simulink model "sampleModel2120"  (R2021a)
settings: Solver=VariableStepAuto  StartTime=0.0  StopTime=10.0  RelTol=1e-3
undefined symbols (not defined in the file or in its folder): DiscIntNeverNeededParam, magnitude, Newton, Raphson
libraries: simulink x67, pid_lib x12
(part 1 of 2)
settings Model: Creator=lenovo  LastModifiedBy=lenovo

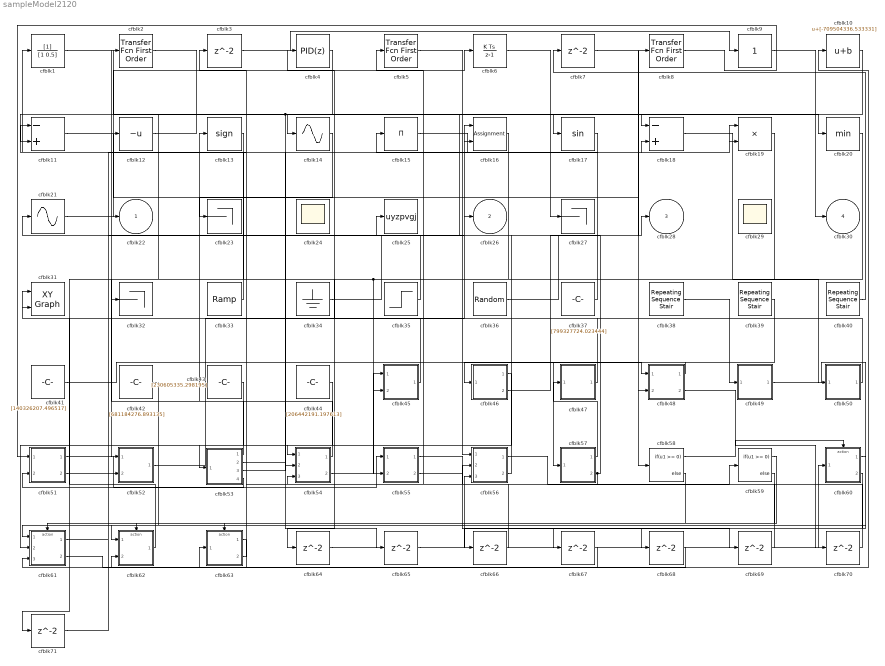
== system sampleModel2120 ==
  cfblk1 : DiscreteFilter  SampleTime=1
  cfblk10 : Bias  Bias=[-709504336.533331]
  cfblk11 : Sum  Inputs=-+
  cfblk12 : UnaryMinus
  cfblk13 : Signum
  cfblk14 : Sin  TimeSource=Use external signal  SampleTime=0
  cfblk15 : Product  Inputs=*
  cfblk16 : Assignment  DiagnosticForDimensions=Warning  IndexOptions=Index vector (dialog)  Indices=1  OutputSizes=1
  cfblk17 : Trigonometry
  cfblk18 : Sum  Inputs=-+
  cfblk19 : Product  Inputs=**
  cfblk2 : simulink/Discrete/Transfer Fcn First Order  PoleZ=0.95  ICPrevOutput=0.0  DoSatur=off
  cfblk20 : MinMax
  cfblk21 : Sin  TimeSource=Use external signal  SampleTime=0
  cfblk23 : Terminator
  cfblk24 : Scope
      settings: Floating=on
  cfblk25 : ToWorkspace  VariableName=uyzpvgj  SaveFormat=Timeseries  SampleTime=-1
  cfblk27 : Terminator
  cfblk29 : Scope
      settings: Floating=on
  cfblk{3,7,64..71} (10 alike) : Delay  SampleTime=1
  cfblk31 : simulink/Sinks/XY Graph  xmin=-1  xmax=1  ymin=-1  ymax=1  st=-1
  cfblk32 : Terminator
  cfblk33 : simulink/Sources/Ramp  slope=[-9170.423728]  start=[47.124759]  InitialOutput=[-914026.200250]
  cfblk34 : Ground
  cfblk35 : Step  Time=[9.000000]  Before=[-795213372.799819]  After=[478961987.281532]  SampleTime=0
  cfblk36 : RandomNumber  Mean=[10617.420643]  Variance=[21176.794349]  Seed=[230646429.000000]  SampleTime=0.1
  cfblk37 : Constant  Value=[799327724.023444]  SampleTime=1
  cfblk38 : simulink/Sources/Repeating Sequence Stair  OutValues=[-433408772.823916, -415254257.712957]  tsamp=-1  OutMin=[]  OutMax=[]  OutDataTypeStr=double  OutputDataTypeScalingMode=double  OutDataType=fixdt(0,8)  ConRadixGroup=Best Precision: Vector-wise  OutScaling=2^-12
  cfblk39 : simulink/Sources/Repeating Sequence Stair  OutValues=[-289850517.751217, -807875800.203243]  tsamp=-1  OutMin=[]  OutMax=[]  OutDataTypeStr=double  OutputDataTypeScalingMode=double  OutDataType=fixdt(0,8)  ConRadixGroup=Best Precision: Vector-wise  OutScaling=2^-12
  cfblk4 : pid_lib/PID Controller  Controller=PID  Form=Parallel  TimeDomain=Discrete-time  UseExternalTs=off  SampleTime=1  IntegratorMethod=Forward Euler  FilterMethod=Forward Euler  ControllerParametersSource=internal  P=1  I=1  D=0  UseFilter=on  N=100  TunerSelectOption=Transfer Function Based (PID Tuner App)  InitialConditionSource=internal  InitialConditionForIntegrator=0  InitialConditionForFilter=0  DifferentiatorICPrevScaledInput=0  ExternalReset=none  TrackingMode=off  Kt=1  LimitOutput=off  SatLimitsSource=internal  UpperSaturationLimit=inf  LowerSaturationLimit=-inf  LinearizeAsGain=off  AntiWindupMode=none  Kb=1  POutMin=[]  POutMax=[]  IOutMin=[]  IOutMax=[]  DOutMin=[]  DOutMax=[]  NOutMin=[]  NOutMax=[]  SumOutMin=[]  SumOutMax=[]  SaturationOutMin=[]  SaturationOutMax=[]  PParamMin=[]  PParamMax=[]  IParamMin=[]  IParamMax=[]  DParamMin=[]  DParamMax=[]  NParamMin=[]  NParamMax=[]  KbParamMin=[]  KbParamMax=[]  KtParamMin=[]  KtParamMax=[]  KbOutMin=[]  KbOutMax=[]  KtOutMin=[]  KtOutMax=[]  IntegratorOutMin=[]  IntegratorOutMax=[]  FilterOutMin=[]  FilterOutMax=[]  SumI1OutMin=[]  SumI1OutMax=[]  SumI2OutMin=[]  SumI2OutMax=[]  SumI3OutMin=[]  SumI3OutMax=[]  SumI4OutMin=[]  SumI4OutMax=[]  SumDOutMin=[]  SumDOutMax=[]  DifferentiatorOutMin=[]  DifferentiatorOutMax=[]  FilterDiffOutCoefMin=[]  FilterDiffOutCoefMax=[]  ReciprocalOutMin=[]  ReciprocalOutMax=[]  SumDenOutMin=[]  SumDenOutMax=[]  SumNumOutMin=[]  SumNumOutMax=[]  DivideOutMin=[]  DivideOutMax=[]  UdiffTsProdOutMin=[]  UdiffTsProdOutMax=[]  NTsProdOutMin=[]  NTsProdOutMax=[]  UintegralTsProdOutMin=[]  UintegralTsProdOutMax=[]  UngainTsProdOutMin=[]  UngainTsProdOutMax=[]  IntegratorContinuousStateAttributes=''  IntegratorStateMustResolveToSignalObject=off  IntegratorRTWStateStorageClass=Auto  FilterContinuousStateAttributes=''  FilterStateMustResolveToSignalObject=off  FilterRTWStateStorageClass=Auto  ParallelPVariant=InternalParameters  IdealPVariant=Disabled  IVariant=InternalParameters  DVariant=InternalParameters  IntegratorVariant=Discrete  SatVariant=Disabled  AWVariant=Passthrough  PCopyVariant=Disabled  TRVariant=Disabled  FdbkBlocksVariant=Forward  IdealPFdbkVariant=Disabled  SatFdbkVariant=Disabled  DerivativeFilterVariant=ForwardEulerFilter  NVariant=InternalParameters  NCopyVariant=Disabled  FilterICVariant=InternalICsFilter  IntegratorICVariant=InternalICs  ExternalResetVariant=Disabled  TRSumVariant=Passthrough  SumFdbkVariant=Disabled  SumVariant=Sum_PID  TsampFilterVariant=InternalTs  TsampNgainVariant=Passthrough  TsampIntegralVariant=Passthrough  ExternalSaturationOutDataTypeStr=Inherit: Same as second input
  cfblk40 : simulink/Sources/Repeating Sequence Stair  OutValues=[599228246.238422, -891664695.317547]  tsamp=-1  OutMin=[]  OutMax=[]  OutDataTypeStr=double  OutputDataTypeScalingMode=double  OutDataType=fixdt(0,8)  ConRadixGroup=Best Precision: Vector-wise  OutScaling=2^-12
  cfblk41 : Constant  Value=[140326207.496517]  SampleTime=1
  cfblk42 : Constant  Value=[681184276.893135]  SampleTime=1
  cfblk43 : Constant  Value=[230605335.298195]  SampleTime=1
  cfblk44 : Constant  Value=[206442191.197613]  SampleTime=1
  cfblk45 : Subsystem
  cfblk46 : Subsystem
  cfblk47 : Subsystem
  cfblk48 : Subsystem
  cfblk49 : Subsystem
  cfblk5 : simulink/Discrete/Transfer Fcn First Order  PoleZ=0.95  ICPrevOutput=0.0  DoSatur=off
  cfblk50 : Subsystem
  cfblk51 : Subsystem
  cfblk52 : Subsystem
  cfblk53 : Subsystem
  cfblk54 : Subsystem
  cfblk55 : Subsystem
  cfblk56 : Subsystem
  cfblk57 : Subsystem
  cfblk58 : If  IfExpression=u1 >= 0  SampleTime=1
  cfblk59 : If  IfExpression=u1 >= 0  SampleTime=1
  cfblk6 : DiscreteIntegrator  ICPrevOutput=DiscIntNeverNeededParam  ICPrevScaledInput=DiscIntNeverNeededParam
  cfblk60 : Subsystem  TreatAsAtomicUnit=on
  cfblk61 : Subsystem  TreatAsAtomicUnit=on
  cfblk62 : Subsystem  TreatAsAtomicUnit=on
  cfblk63 : Subsystem  TreatAsAtomicUnit=on
  cfblk8 : simulink/Discrete/Transfer Fcn First Order  PoleZ=0.95  ICPrevOutput=0.0  DoSatur=off
  cfblk9 : simulink/Math Operations/Slider Gain  gain=1  low=0  high=2
  cfblk22 : Outport
  cfblk26 : Outport  Port=2
  cfblk28 : Outport  Port=3
  cfblk30 : Outport  Port=4
  wires:
  cfblk1/1 -> cfblk14/1
  cfblk33/1 -> cfblk1/1
  cfblk52/1(cfblk2) -> cfblk16/1
  cfblk3/1 -> cfblk9/1
  cfblk49/1(cfblk2) -> cfblk61/1(cfblk1)
  cfblk44/1 -> cfblk54/1(cfblk1)
  cfblk21/1 -> cfblk6/1
  cfblk39/1 -> cfblk57/1(cfblk1)
  cfblk51/1(cfblk2) -> cfblk55/1(cfblk1)
  cfblk53/1(cfblk2) -> cfblk2/1
  cfblk45/1(cfblk2) -> cfblk31/1
  cfblk34/1 -> cfblk20/1
  cfblk8/1 -> cfblk51/1(cfblk1)
  cfblk54/1(cfblk2) -> cfblk13/1
  cfblk43/1 -> cfblk61/2(cfblk12)
  cfblk13/1 -> cfblk52/1(cfblk1)
  cfblk40/1 -> cfblk7/1
  cfblk18/1 -> cfblk50/1(cfblk1)
  cfblk12/1 -> cfblk17/1
  cfblk57/1(cfblk2) -> cfblk47/1(cfblk1)
  cfblk37/1 -> cfblk15/1
  cfblk9/1 -> cfblk30/1
  cfblk35/1 -> cfblk21/1
  cfblk14/1 -> cfblk23/1
  cfblk38/1 -> cfblk49/1(cfblk1)
  cfblk41/1 -> cfblk48/1(cfblk1)
  cfblk51/2(cfblk12) -> cfblk26/1
  cfblk57/2(cfblk17) -> cfblk22/1, cfblk54/3(cfblk11)
  cfblk46/1(cfblk2) -> cfblk53/1(cfblk1)
  cfblk7/1 -> cfblk58/1
  cfblk46/2(cfblk8) -> cfblk28/1
  cfblk42/1 -> cfblk62/1(cfblk1)
  cfblk61/1(cfblk2) -> cfblk19/1
  cfblk62/1(cfblk2) -> cfblk31/2
  cfblk16/1 -> cfblk45/2(cfblk15), cfblk71/1
  cfblk6/1 -> cfblk27/1
  cfblk50/1(cfblk2) -> cfblk3/1
  cfblk47/1(cfblk2) -> cfblk4/1
  cfblk36/1 -> cfblk8/1
  cfblk5/1 -> cfblk56/1(cfblk1)
  cfblk4/1 -> cfblk32/1
  cfblk15/1 -> cfblk19/2
  cfblk17/1 -> cfblk16/2
  cfblk61/2(cfblk14) -> cfblk10/1
  cfblk11/1 -> cfblk48/2(cfblk13)
  cfblk20/1 -> cfblk55/2(cfblk10)
  cfblk2/1 -> cfblk18/1
  cfblk53/3(cfblk6) -> cfblk18/2
  cfblk56/1(cfblk2) -> cfblk59/1
  cfblk10/1 -> cfblk11/2, cfblk54/2(cfblk10)
  cfblk63/1(cfblk2) -> cfblk61/3(cfblk13)
  cfblk56/2(cfblk12) -> cfblk25/1
  cfblk53/4(cfblk7) -> cfblk51/2(cfblk11)
  cfblk48/1(cfblk2) -> cfblk46/1(cfblk1)
  cfblk63/2(cfblk8) -> cfblk12/1
  cfblk54/2(cfblk12) -> cfblk45/1(cfblk1)
  cfblk58/1 -> cfblk60/Action
  cfblk58/2 -> cfblk61/Action
  cfblk59/1 -> cfblk62/Action
  cfblk59/2 -> cfblk63/Action
  cfblk19/1 -> cfblk64/1
  cfblk64/1 -> cfblk56/3(cfblk11)
  cfblk53/2(cfblk5) -> cfblk65/1
  cfblk65/1 -> cfblk60/1(cfblk1)
  cfblk60/1(cfblk2) -> cfblk66/1
  cfblk66/1 -> cfblk11/1
  cfblk60/2(cfblk14) -> cfblk67/1
  cfblk67/1 -> cfblk62/2(cfblk13)
  cfblk55/1(cfblk2) -> cfblk68/1
  cfblk68/1 -> cfblk63/1(cfblk1)
  cfblk55/2(cfblk11) -> cfblk69/1
  cfblk69/1 -> cfblk5/1
  cfblk48/2(cfblk14) -> cfblk70/1
  cfblk70/1 -> cfblk56/2(cfblk10)
  cfblk71/1 -> cfblk52/2(cfblk15)

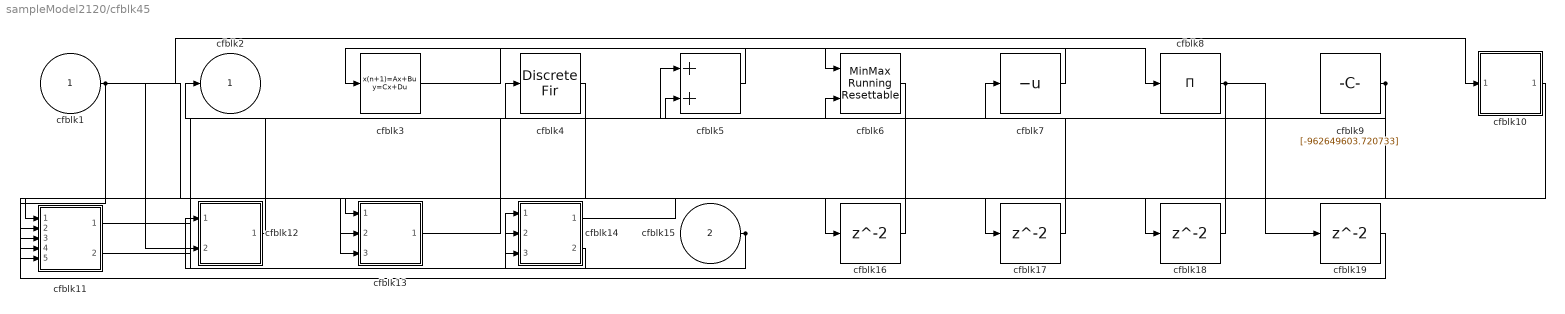
== system sampleModel2120/cfblk45 ==
  cfblk1 : Inport
  cfblk15 : Inport  Port=2
  cfblk10 : Subsystem
  cfblk11 : Subsystem
  cfblk12 : Subsystem
  cfblk13 : Subsystem
  cfblk14 : Subsystem
  cfblk{16..19} (4 alike) : Delay  SampleTime=1
  cfblk3 : DiscreteStateSpace
  cfblk4 : DiscreteFir  SampleTime=1
  cfblk5 : Sum
  cfblk6 : simulink/Math Operations/MinMax Running Resettable  Function=min  vinit=0.0
  cfblk7 : UnaryMinus
  cfblk8 : Product  Inputs=*
  cfblk9 : Constant  Value=[-962649603.720733]  SampleTime=1
  cfblk2 : Outport
  wires:
  cfblk5/1 -> cfblk3/1
  cfblk12/1(cfblk2) -> cfblk2/1
  cfblk7/1 -> cfblk6/1
  cfblk1/1 -> cfblk10/1(cfblk1), cfblk11/3(cfblk7), cfblk12/2(cfblk11), cfblk13/3(cfblk12)
  cfblk11/1(cfblk2) -> cfblk14/1(cfblk1)
  cfblk9/1 -> cfblk4/1, cfblk11/5(cfblk9)
  cfblk8/1 -> cfblk17/1, cfblk18/1, cfblk19/1
  cfblk3/1 -> cfblk8/1
  cfblk4/1 -> cfblk11/1(cfblk1)
  cfblk13/1(cfblk2) -> cfblk7/1
  cfblk6/1 -> cfblk11/2(cfblk6)
  cfblk10/1(cfblk2) -> cfblk13/1(cfblk1)
  cfblk11/2(cfblk10) -> cfblk5/2
  cfblk15/1 -> cfblk14/2(cfblk7), cfblk14/3(cfblk8)
  cfblk14/2(cfblk9) -> cfblk12/1(cfblk1)
  cfblk14/1(cfblk2) -> cfblk16/1
  cfblk16/1 -> cfblk6/2
  cfblk17/1 -> cfblk5/1
  cfblk18/1 -> cfblk13/2(cfblk11)
  cfblk19/1 -> cfblk11/4(cfblk8)

== system sampleModel2120/cfblk46 ==
  cfblk1 : Inport
  cfblk10 : Delay  SampleTime=1
  cfblk11 : Delay  SampleTime=1
  cfblk3 : Signum
  cfblk4 : PermuteDimensions
  cfblk5 : simulink/Math Operations/MinMax Running Resettable  Function=min  vinit=0.0
  cfblk6 : Reshape
  cfblk7 : Subsystem
  cfblk9 : Delay  SampleTime=1
  cfblk2 : Outport
  cfblk8 : Outport  Port=2
  wires:
  cfblk5/1 -> cfblk8/1, cfblk10/1
  cfblk7/1(cfblk2) -> cfblk4/1
  cfblk3/1 -> cfblk2/1, cfblk5/2, cfblk11/1
  cfblk1/1 -> cfblk7/4(cfblk16)
  cfblk7/2(cfblk17) -> cfblk6/1, cfblk3/1
  cfblk6/1 -> cfblk5/1
  cfblk4/1 -> cfblk9/1
  cfblk9/1 -> cfblk7/1(cfblk1)
  cfblk10/1 -> cfblk7/2(cfblk14)
  cfblk11/1 -> cfblk7/3(cfblk15)

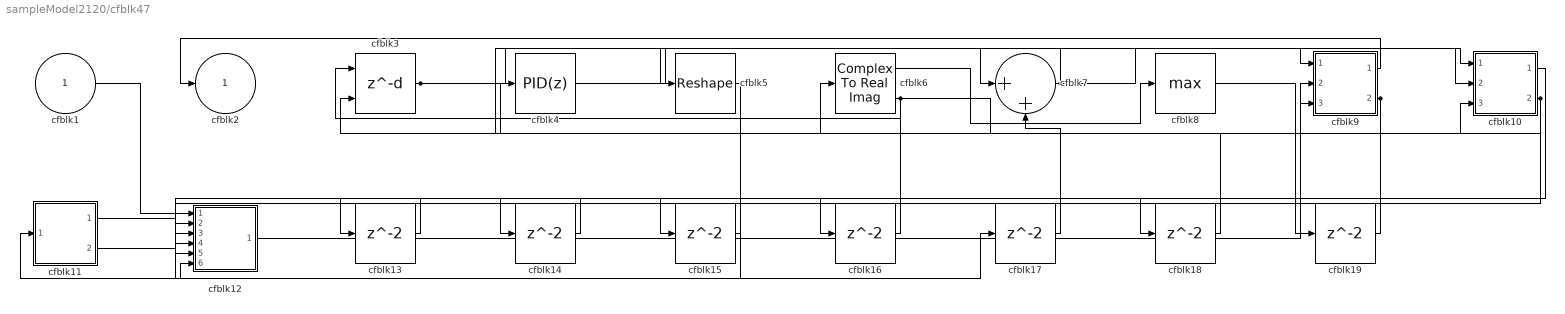
== system sampleModel2120/cfblk47 ==
  cfblk1 : Inport
  cfblk10 : Subsystem
  cfblk11 : Subsystem
  cfblk12 : Subsystem
  cfblk{13..19} (7 alike) : Delay  SampleTime=1
  cfblk3 : Delay  DelayLengthSource=Input port  SampleTime=1
      settings: InputPortMap=u0,p1
  cfblk4 : pid_lib/PID Controller  Controller=PID  Form=Parallel  TimeDomain=Discrete-time  UseExternalTs=off  SampleTime=1  IntegratorMethod=Forward Euler  FilterMethod=Forward Euler  ControllerParametersSource=internal  P=1  I=1  D=0  UseFilter=on  N=100  TunerSelectOption=Transfer Function Based (PID Tuner App)  InitialConditionSource=internal  InitialConditionForIntegrator=0  InitialConditionForFilter=0  DifferentiatorICPrevScaledInput=0  ExternalReset=none  TrackingMode=off  Kt=1  LimitOutput=off  SatLimitsSource=internal  UpperSaturationLimit=inf  LowerSaturationLimit=-inf  LinearizeAsGain=off  AntiWindupMode=none  Kb=1  POutMin=[]  POutMax=[]  IOutMin=[]  IOutMax=[]  DOutMin=[]  DOutMax=[]  NOutMin=[]  NOutMax=[]  SumOutMin=[]  SumOutMax=[]  SaturationOutMin=[]  SaturationOutMax=[]  PParamMin=[]  PParamMax=[]  IParamMin=[]  IParamMax=[]  DParamMin=[]  DParamMax=[]  NParamMin=[]  NParamMax=[]  KbParamMin=[]  KbParamMax=[]  KtParamMin=[]  KtParamMax=[]  KbOutMin=[]  KbOutMax=[]  KtOutMin=[]  KtOutMax=[]  IntegratorOutMin=[]  IntegratorOutMax=[]  FilterOutMin=[]  FilterOutMax=[]  SumI1OutMin=[]  SumI1OutMax=[]  SumI2OutMin=[]  SumI2OutMax=[]  SumI3OutMin=[]  SumI3OutMax=[]  SumI4OutMin=[]  SumI4OutMax=[]  SumDOutMin=[]  SumDOutMax=[]  DifferentiatorOutMin=[]  DifferentiatorOutMax=[]  FilterDiffOutCoefMin=[]  FilterDiffOutCoefMax=[]  ReciprocalOutMin=[]  ReciprocalOutMax=[]  SumDenOutMin=[]  SumDenOutMax=[]  SumNumOutMin=[]  SumNumOutMax=[]  DivideOutMin=[]  DivideOutMax=[]  UdiffTsProdOutMin=[]  UdiffTsProdOutMax=[]  NTsProdOutMin=[]  NTsProdOutMax=[]  UintegralTsProdOutMin=[]  UintegralTsProdOutMax=[]  UngainTsProdOutMin=[]  UngainTsProdOutMax=[]  IntegratorContinuousStateAttributes=''  IntegratorStateMustResolveToSignalObject=off  IntegratorRTWStateStorageClass=Auto  FilterContinuousStateAttributes=''  FilterStateMustResolveToSignalObject=off  FilterRTWStateStorageClass=Auto  ParallelPVariant=InternalParameters  IdealPVariant=Disabled  IVariant=InternalParameters  DVariant=InternalParameters  IntegratorVariant=Discrete  SatVariant=Disabled  AWVariant=Passthrough  PCopyVariant=Disabled  TRVariant=Disabled  FdbkBlocksVariant=Forward  IdealPFdbkVariant=Disabled  SatFdbkVariant=Disabled  DerivativeFilterVariant=ForwardEulerFilter  NVariant=InternalParameters  NCopyVariant=Disabled  FilterICVariant=InternalICsFilter  IntegratorICVariant=InternalICs  ExternalResetVariant=Disabled  TRSumVariant=Passthrough  SumFdbkVariant=Disabled  SumVariant=Sum_PID  TsampFilterVariant=InternalTs  TsampNgainVariant=Passthrough  TsampIntegralVariant=Passthrough  ExternalSaturationOutDataTypeStr=Inherit: Same as second input
  cfblk5 : Reshape
  cfblk6 : ComplexToRealImag
  cfblk7 : Sum  Inputs=|++
  cfblk8 : MinMax  Function=max
  cfblk9 : Subsystem
  cfblk2 : Outport
  wires:
  cfblk3/1 -> cfblk7/1, cfblk10/2(cfblk13), cfblk10/3(cfblk14)
  cfblk9/1(cfblk2) -> cfblk2/1
  cfblk5/1 -> cfblk11/1(cfblk1)
  cfblk6/1 -> cfblk8/1
  cfblk4/1 -> cfblk9/1(cfblk1)
  cfblk10/2(cfblk15) -> cfblk4/1, cfblk12/5(cfblk14)
  cfblk1/1 -> cfblk12/1(cfblk1)
  cfblk7/1 -> cfblk5/1, cfblk10/1(cfblk1)
  cfblk6/2 -> cfblk9/2(cfblk12), cfblk12/4(cfblk13)
  cfblk9/2(cfblk14) -> cfblk13/1, cfblk14/1, cfblk15/1
  cfblk12/1(cfblk2) -> cfblk9/3(cfblk13)
  cfblk13/1 -> cfblk12/2(cfblk11)
  cfblk14/1 -> cfblk12/3(cfblk12)
  cfblk15/1 -> cfblk12/6(cfblk15)
  cfblk11/1(cfblk2) -> cfblk16/1
  cfblk16/1 -> cfblk3/1
  cfblk11/2(cfblk10) -> cfblk17/1
  cfblk17/1 -> cfblk7/2
  cfblk10/1(cfblk2) -> cfblk18/1
  cfblk18/1 -> cfblk3/2
  cfblk8/1 -> cfblk19/1
  cfblk19/1 -> cfblk6/1

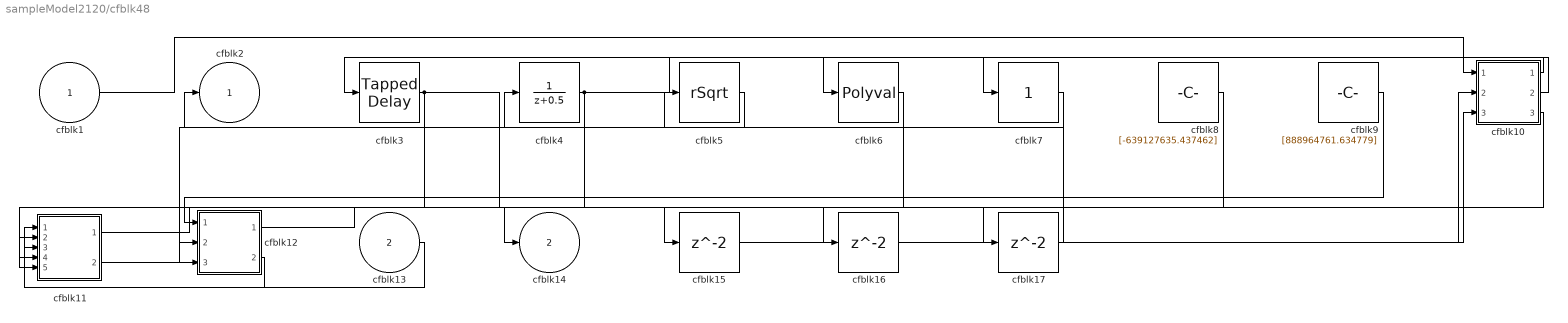
== system sampleModel2120/cfblk48 ==
  cfblk1 : Inport
  cfblk13 : Inport  Port=2
  cfblk10 : Subsystem
  cfblk11 : Subsystem
  cfblk12 : Subsystem
  cfblk15 : Delay  SampleTime=1
  cfblk16 : Delay  SampleTime=1
  cfblk17 : Delay  SampleTime=1
  cfblk3 : simulink/Discrete/Tapped Delay  vinit=0.0  samptime=-1  NumDelays=1  DelayOrder=Oldest  includeCurrent=off
  cfblk4 : DiscreteTransferFcn  SampleTime=1
  cfblk5 : Sqrt  Operator=rSqrt  AlgorithmType=Newton-Raphson  SaturateOnIntegerOverflow=on
  cfblk6 : Polyval  Coefs=[ +2.081618890e-019, -1.441693666e-014, +4.719686976e-010, -8.536869453e-006, +1.621573104e-001, -8.087801117e+001 ]
  cfblk7 : simulink/Math Operations/Slider Gain  gain=1  low=0  high=2
  cfblk8 : Constant  Value=[-639127635.437462]  SampleTime=1
  cfblk9 : Constant  Value=[888964761.634779]  SampleTime=1
  cfblk2 : Outport
  cfblk14 : Outport  Port=2
  wires:
  cfblk4/1 -> cfblk7/1, cfblk11/5(cfblk10)
  cfblk5/1 -> cfblk2/1
  cfblk11/1(cfblk2) -> cfblk14/1
  cfblk9/1 -> cfblk12/1(cfblk1)
  cfblk13/1 -> cfblk11/1(cfblk1)
  cfblk3/1 -> cfblk11/2(cfblk7), cfblk16/1
  cfblk11/2(cfblk11) -> cfblk5/1
  cfblk8/1 -> cfblk12/2(cfblk8)
  cfblk1/1 -> cfblk10/1(cfblk1)
  cfblk6/1 -> cfblk12/3(cfblk9)
  cfblk12/2(cfblk10) -> cfblk11/3(cfblk8)
  cfblk10/1(cfblk2) -> cfblk6/1
  cfblk10/2(cfblk16) -> cfblk3/1
  cfblk10/3(cfblk17) -> cfblk11/4(cfblk9)
  cfblk12/1(cfblk2) -> cfblk15/1
  cfblk15/1 -> cfblk10/2(cfblk14)
  cfblk16/1 -> cfblk10/3(cfblk15)
  cfblk7/1 -> cfblk17/1
  cfblk17/1 -> cfblk4/1

== system sampleModel2120/cfblk49 ==
  cfblk1 : Inport
  cfblk{8..12} (5 alike) : Delay  SampleTime=1
  cfblk3 : Polyval  Coefs=[ +2.081618890e-019, -1.441693666e-014, +4.719686976e-010, -8.536869453e-006, +1.621573104e-001, -8.087801117e+001 ]
  cfblk4 : Reshape
  cfblk5 : Subsystem
  cfblk6 : Subsystem
  cfblk7 : Subsystem
  cfblk2 : Outport
  wires:
  cfblk3/1 -> cfblk4/1, cfblk10/1
  cfblk4/1 -> cfblk8/1, cfblk9/1
  cfblk1/1 -> cfblk6/2(cfblk11)
  cfblk6/1(cfblk2) -> cfblk3/1
  cfblk5/1(cfblk2) -> cfblk2/1, cfblk11/1, cfblk12/1
  cfblk7/1(cfblk2) -> cfblk5/1(cfblk1)
  cfblk6/2(cfblk15) -> cfblk7/1(cfblk1)
  cfblk6/3(cfblk16) -> cfblk5/2(cfblk7)
  cfblk6/4(cfblk17) -> cfblk7/2(cfblk12)
  cfblk8/1 -> cfblk6/1(cfblk1)
  cfblk9/1 -> cfblk6/5(cfblk14)
  cfblk10/1 -> cfblk6/3(cfblk12)
  cfblk11/1 -> cfblk6/4(cfblk13)
  cfblk12/1 -> cfblk7/3(cfblk13)

== system sampleModel2120/cfblk50 ==
  cfblk1 : Inport
  cfblk3 : simulink/Discrete/Difference  ICPrevInput=0.0  OutMin=[]  OutMax=[]  OutDataTypeStr=Inherit: Inherit via back propagation  OutDataType=fixdt(1, 16)  OutScaling=2^-10  DoSatur=off
  cfblk4 : simulink/Discrete/Transfer Fcn Real Zero  ZeroZ=0.75  ICPrevInput=0.0  DoSatur=off
      settings: SourceProductBaseCode=SL
  cfblk5 : simulink/Discrete/Transfer Fcn First Order  PoleZ=0.95  ICPrevOutput=0.0  DoSatur=off
  cfblk6 : simulink/Discrete/Difference  ICPrevInput=0.0  OutMin=[]  OutMax=[]  OutDataTypeStr=Inherit: Inherit via back propagation  OutDataType=fixdt(1, 16)  OutScaling=2^-10  DoSatur=off
  cfblk7 : Sin  TimeSource=Use external signal  SampleTime=0
  cfblk2 : Outport
  wires:
  cfblk3/1 -> cfblk7/1
  cfblk7/1 -> cfblk4/1
  cfblk1/1 -> cfblk5/1
  cfblk5/1 -> cfblk3/1
  cfblk4/1 -> cfblk6/1
  cfblk6/1 -> cfblk2/1

== system sampleModel2120/cfblk51 ==
  cfblk1 : Inport
  cfblk11 : Inport  Port=2
  cfblk10 : Subsystem
  cfblk{13..16} (4 alike) : Delay  SampleTime=1
  cfblk3 : Delay  ShowEnablePort=on  SampleTime=1
      settings: InputPortMap=u0,e6
  cfblk4 : Assignment  DiagnosticForDimensions=Warning  IndexOptions=Index vector (dialog)  Indices=1  OutputSizes=1
  cfblk5 : Rounding
  cfblk6 : Rounding
  cfblk7 : Abs
  cfblk8 : Constant  Value=[-895751787.205056]  SampleTime=1
  cfblk9 : Subsystem
  cfblk2 : Outport
  cfblk12 : Outport  Port=2
  wires:
  cfblk5/1 -> cfblk4/1, cfblk15/1, cfblk16/1
  cfblk7/1 -> cfblk12/1
  cfblk11/1 -> cfblk10/1(cfblk1), cfblk9/5(cfblk12)
  cfblk1/1 -> cfblk6/1, cfblk10/6(cfblk15)
  cfblk6/1 -> cfblk4/2, cfblk10/4(cfblk13)
  cfblk10/1(cfblk2) -> cfblk2/1
  cfblk9/1(cfblk2) -> cfblk3/1
  cfblk4/1 -> cfblk7/1
  cfblk3/1 -> cfblk13/1, cfblk14/1
  cfblk10/2(cfblk16) -> cfblk9/2(cfblk9)
  cfblk8/1 -> cfblk9/3(cfblk10), cfblk10/3(cfblk12), cfblk3/2
  cfblk9/2(cfblk14) -> cfblk5/1
  cfblk10/3(cfblk17) -> cfblk9/4(cfblk11)
  cfblk13/1 -> cfblk9/1(cfblk1)
  cfblk14/1 -> cfblk9/6(cfblk13)
  cfblk15/1 -> cfblk10/2(cfblk11)
  cfblk16/1 -> cfblk10/5(cfblk14)

== system sampleModel2120/cfblk52 ==
  cfblk1 : Inport
  cfblk15 : Inport  Port=2
  cfblk10 : Math  Operator=pow  SaturateOnIntegerOverflow=on
  cfblk11 : simulink/Math Operations/Slider Gain  gain=1  low=0  high=2
  cfblk12 : Abs
  cfblk13 : Constant  Value=[906795695.225811]  SampleTime=1
  cfblk14 : Subsystem
  cfblk16 : Delay  SampleTime=1
  cfblk3 : DiscreteFir  SampleTime=1
  cfblk4 : DiscreteStateSpace
  cfblk5 : DiscreteStateSpace
  cfblk6 : DiscreteTransferFcn  SampleTime=1
  cfblk7 : DiscreteFir  SampleTime=1
  cfblk8 : DiscreteIntegrator  ICPrevOutput=DiscIntNeverNeededParam  ICPrevScaledInput=DiscIntNeverNeededParam
  cfblk9 : Sum  Inputs=-+
  cfblk2 : Outport
  wires:
  cfblk4/1 -> cfblk12/1
  cfblk12/1 -> cfblk6/1, cfblk10/2
  cfblk13/1 -> cfblk11/1
  cfblk14/1(cfblk2) -> cfblk5/1
  cfblk1/1 -> cfblk14/1(cfblk1)
  cfblk15/1 -> cfblk8/1, cfblk10/1
  cfblk10/1 -> cfblk14/2(cfblk14)
  cfblk3/1 -> cfblk2/1
  cfblk8/1 -> cfblk9/1, cfblk14/5(cfblk17)
  cfblk7/1 -> cfblk3/1
  cfblk6/1 -> cfblk9/2, cfblk16/1
  cfblk11/1 -> cfblk14/3(cfblk15)
  cfblk5/1 -> cfblk7/1
  cfblk9/1 -> cfblk14/4(cfblk16)
  cfblk16/1 -> cfblk4/1

== system sampleModel2120/cfblk53 ==
  cfblk1 : Inport
  cfblk3 : Subsystem
  cfblk4 : Subsystem
  cfblk2 : Outport
  cfblk5 : Outport  Port=2
  cfblk6 : Outport  Port=3
  cfblk7 : Outport  Port=4
  wires:
  cfblk1/1 -> cfblk2/1, cfblk3/1(cfblk1), cfblk3/2(cfblk9)
  cfblk3/1(cfblk2) -> cfblk5/1
  cfblk3/2(cfblk10) -> cfblk4/1(cfblk1)
  cfblk3/3(cfblk11) -> cfblk4/2(cfblk8)
  cfblk3/4(cfblk12) -> cfblk4/3(cfblk9)
  cfblk3/5(cfblk13) -> cfblk7/1
  cfblk4/1(cfblk2) -> cfblk6/1

== system sampleModel2120/cfblk54 ==
  cfblk1 : Inport
  cfblk10 : Inport  Port=2
  cfblk11 : Inport  Port=3
  cfblk13 : Delay  SampleTime=1
  cfblk3 : DiscreteFir  SampleTime=1
  cfblk4 : Math  Operator=magnitude^2  SaturateOnIntegerOverflow=on
  cfblk5 : PermuteDimensions
  cfblk6 : Subsystem
  cfblk7 : Subsystem
  cfblk8 : Subsystem
  cfblk9 : Subsystem
  cfblk2 : Outport
  cfblk12 : Outport  Port=2
  wires:
  cfblk9/1(cfblk2) -> cfblk8/1(cfblk1)
  cfblk11/1 -> cfblk7/1(cfblk1)
  cfblk7/1(cfblk2) -> cfblk6/1(cfblk1)
  cfblk3/1 -> cfblk2/1
  cfblk9/2(cfblk8) -> cfblk12/1
  cfblk5/1 -> cfblk4/1
  cfblk10/1 -> cfblk3/1
  cfblk9/3(cfblk9) -> cfblk6/2(cfblk9)
  cfblk4/1 -> cfblk6/3(cfblk10)
  cfblk1/1 -> cfblk9/1(cfblk1)
  cfblk8/1(cfblk2) -> cfblk5/1, cfblk6/4(cfblk11), cfblk6/5(cfblk12)
  cfblk6/1(cfblk2) -> cfblk13/1
  cfblk13/1 -> cfblk9/2(cfblk7)

== system sampleModel2120/cfblk55 ==
  cfblk1 : Inport
  cfblk10 : Inport  Port=2
  cfblk12 : Delay  SampleTime=1
  cfblk13 : Delay  SampleTime=1
  cfblk14 : Delay  SampleTime=1
  cfblk3 : simulink/Discrete/Transfer Fcn First Order  PoleZ=0.95  ICPrevOutput=0.0  DoSatur=off
  cfblk4 : PermuteDimensions
  cfblk5 : Sum  Inputs=+-
  cfblk6 : Product  Inputs=**
  cfblk7 : Subsystem
  cfblk8 : Subsystem
  cfblk9 : Subsystem
  cfblk2 : Outport
  cfblk11 : Outport  Port=2
  wires:
  cfblk3/1 -> cfblk7/1(cfblk1)
  cfblk8/1(cfblk2) -> cfblk6/1
  cfblk5/1 -> cfblk6/2, cfblk3/1
  cfblk10/1 -> cfblk2/1, cfblk7/3(cfblk8)
  cfblk1/1 -> cfblk9/4(cfblk14), cfblk5/2, cfblk7/2(cfblk7)
  cfblk8/2(cfblk12) -> cfblk4/1
  cfblk9/1(cfblk2) -> cfblk8/1(cfblk1)
  cfblk9/2(cfblk15) -> cfblk8/2(cfblk10)
  cfblk9/3(cfblk16) -> cfblk5/1, cfblk8/3(cfblk11)
  cfblk8/3(cfblk13) -> cfblk11/1, cfblk7/4(cfblk9)
  cfblk6/1 -> cfblk12/1
  cfblk12/1 -> cfblk9/3(cfblk13)
  cfblk4/1 -> cfblk13/1
  cfblk13/1 -> cfblk9/2(cfblk12)
  cfblk7/1(cfblk2) -> cfblk14/1
  cfblk14/1 -> cfblk9/1(cfblk1)

== system sampleModel2120/cfblk56 ==
  cfblk1 : Inport
  cfblk10 : Inport  Port=2
  cfblk11 : Inport  Port=3
  cfblk3 : DiscreteFilter  SampleTime=1
  cfblk4 : UnitDelay  HasFrameUpgradeWarning=on
  cfblk5 : simulink/Discrete/Difference  ICPrevInput=0.0  OutMin=[]  OutMax=[]  OutDataTypeStr=Inherit: Inherit via back propagation  OutDataType=fixdt(1, 16)  OutScaling=2^-10  DoSatur=off
  cfblk6 : PermuteDimensions
  cfblk7 : Reshape
  cfblk8 : Constant  Value=[483167932.969646]  SampleTime=1
  cfblk9 : Subsystem
  cfblk2 : Outport
  cfblk12 : Outport  Port=2
  wires:
  cfblk8/1 -> cfblk9/1(cfblk1)
  cfblk5/1 -> cfblk3/1
  cfblk6/1 -> cfblk4/1
  cfblk3/1 -> cfblk2/1
  cfblk4/1 -> cfblk12/1
  cfblk7/1 -> cfblk5/1
  cfblk10/1 -> cfblk6/1
  cfblk11/1 -> cfblk9/2(cfblk8)
  cfblk1/1 -> cfblk9/3(cfblk9)
  cfblk9/1(cfblk2) -> cfblk7/1

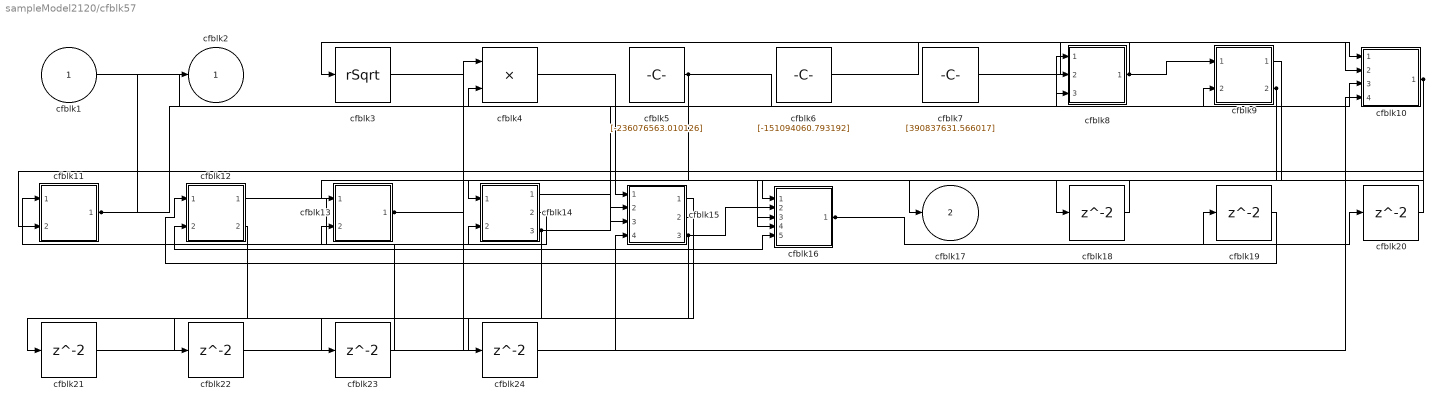
== system sampleModel2120/cfblk57 ==
  cfblk1 : Inport
  cfblk10 : Subsystem
  cfblk11 : Subsystem
  cfblk12 : Subsystem
  cfblk13 : Subsystem
  cfblk14 : Subsystem
  cfblk15 : Subsystem
  cfblk16 : Subsystem
  cfblk{18..24} (7 alike) : Delay  SampleTime=1
  cfblk3 : Sqrt  Operator=rSqrt  AlgorithmType=Newton-Raphson  SaturateOnIntegerOverflow=on
  cfblk4 : Product  Inputs=**
  cfblk5 : Constant  Value=[-236076563.010126]  SampleTime=1
  cfblk6 : Constant  Value=[-151094060.793192]  SampleTime=1
  cfblk7 : Constant  Value=[390837631.566017]  SampleTime=1
  cfblk8 : Subsystem
  cfblk9 : Subsystem
  cfblk2 : Outport
  cfblk17 : Outport  Port=2
  wires:
  cfblk16/1(cfblk2) -> cfblk19/1, cfblk20/1
  cfblk7/1 -> cfblk10/1(cfblk1)
  cfblk15/1(cfblk2) -> cfblk12/2(cfblk8)
  cfblk10/1(cfblk2) -> cfblk11/2(cfblk9), cfblk15/2(cfblk13)
  cfblk6/1 -> cfblk10/2(cfblk6)
  cfblk12/1(cfblk2) -> cfblk14/2(cfblk6)
  cfblk13/1(cfblk2) -> cfblk17/1, cfblk16/5(cfblk16)
  cfblk8/1(cfblk2) -> cfblk9/1(cfblk1), cfblk3/1
  cfblk5/1 -> cfblk13/1(cfblk1), cfblk8/3(cfblk13)
  cfblk1/1 -> cfblk10/3(cfblk7)
  cfblk11/1(cfblk2) -> cfblk4/2, cfblk2/1
  cfblk4/1 -> cfblk15/1(cfblk1)
  cfblk9/2(cfblk7) -> cfblk16/1(cfblk1), cfblk16/3(cfblk14), cfblk16/4(cfblk15)
  cfblk15/3(cfblk17) -> cfblk16/2(cfblk13), cfblk24/1
  cfblk14/1(cfblk2) -> cfblk8/1(cfblk1)
  cfblk14/2(cfblk7) -> cfblk13/2(cfblk7)
  cfblk3/1 -> cfblk9/2(cfblk6)
  cfblk14/3(cfblk8) -> cfblk8/2(cfblk12), cfblk21/1
  cfblk9/1(cfblk2) -> cfblk18/1
  cfblk18/1 -> cfblk14/1(cfblk1)
  cfblk19/1 -> cfblk12/1(cfblk1)
  cfblk20/1 -> cfblk15/3(cfblk14)
  cfblk21/1 -> cfblk15/4(cfblk15)
  cfblk12/2(cfblk9) -> cfblk22/1
  cfblk22/1 -> cfblk4/1
  cfblk15/2(cfblk16) -> cfblk23/1
  cfblk23/1 -> cfblk11/1(cfblk1)
  cfblk24/1 -> cfblk10/4(cfblk8)

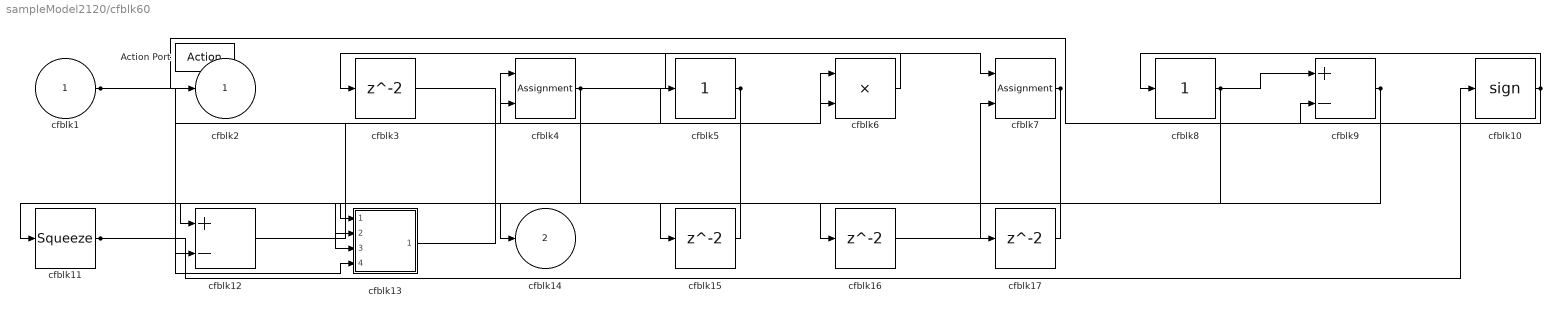
== system sampleModel2120/cfblk60 ==
  cfblk1 : Inport
  Action Port : ActionPort  ActionPortLabel=if(u1 >= 0)
  cfblk10 : Signum
  cfblk11 : Squeeze
  cfblk12 : Sum  Inputs=+-
  cfblk13 : Subsystem
  cfblk{3,15..17} (4 alike) : Delay
  cfblk4 : Assignment  DiagnosticForDimensions=Warning  IndexOptions=Index vector (dialog)  Indices=1  OutputSizes=1
  cfblk5 : simulink/Math Operations/Slider Gain  gain=1  low=0  high=2
  cfblk6 : Product
  cfblk7 : Assignment  DiagnosticForDimensions=Warning  IndexOptions=Index vector (dialog)  Indices=1  OutputSizes=1
  cfblk8 : simulink/Math Operations/Slider Gain  gain=1  low=0  high=2
  cfblk9 : Sum  Inputs=+-
  cfblk2 : Outport
  cfblk14 : Outport  Port=2
  wires:
  cfblk7/1 -> cfblk11/1, cfblk13/2(cfblk7)
  cfblk11/1 -> cfblk10/1, cfblk6/2, cfblk13/4(cfblk9)
  cfblk10/1 -> cfblk8/1, cfblk9/2
  cfblk5/1 -> cfblk14/1, cfblk12/2
  cfblk13/1(cfblk2) -> cfblk6/1
  cfblk4/1 -> cfblk7/1, cfblk13/3(cfblk8)
  cfblk12/1 -> cfblk4/1
  cfblk9/1 -> cfblk2/1, cfblk15/1
  cfblk6/1 -> cfblk3/1
  cfblk1/1 -> cfblk5/1, cfblk13/1(cfblk1)
  cfblk8/1 -> cfblk9/1, cfblk16/1
  cfblk15/1 -> cfblk4/2
  cfblk16/1 -> cfblk7/2
  cfblk3/1 -> cfblk17/1
  cfblk17/1 -> cfblk12/1

== system sampleModel2120/cfblk61 ==
  cfblk1 : Inport
  cfblk12 : Inport  Port=2
  cfblk13 : Inport  Port=3
  Action Port : ActionPort  ActionPortLabel=else
  cfblk10 : Subsystem
  cfblk11 : Subsystem
  cfblk15 : Delay
  cfblk3 : Delay  DelayLengthSource=Input port
      settings: InputPortMap=u0,p1
  cfblk4 : Delay
  cfblk5 : simulink/Math Operations/Slider Gain  gain=1  low=0  high=2
  cfblk6 : Sqrt  SaturateOnIntegerOverflow=on
  cfblk7 : Constant  Value=[999796448.984934]  SampleTime=1
  cfblk8 : Constant  Value=[-825546271.964894]  SampleTime=1
  cfblk9 : Constant  Value=[-268532313.679241]  SampleTime=1
  cfblk2 : Outport
  cfblk14 : Outport  Port=2
  wires:
  cfblk11/1(cfblk2) -> cfblk3/2
  cfblk6/1 -> cfblk2/1
  cfblk9/1 -> cfblk6/1
  cfblk3/1 -> cfblk4/1
  cfblk4/1 -> cfblk5/1
  cfblk7/1 -> cfblk14/1
  cfblk11/2(cfblk7) -> cfblk10/1(cfblk1)
  cfblk12/1 -> cfblk10/2(cfblk8)
  cfblk13/1 -> cfblk10/3(cfblk9)
  cfblk8/1 -> cfblk10/4(cfblk10)
  cfblk1/1 -> cfblk11/1(cfblk1)
  cfblk5/1 -> cfblk15/1
  cfblk15/1 -> cfblk3/1

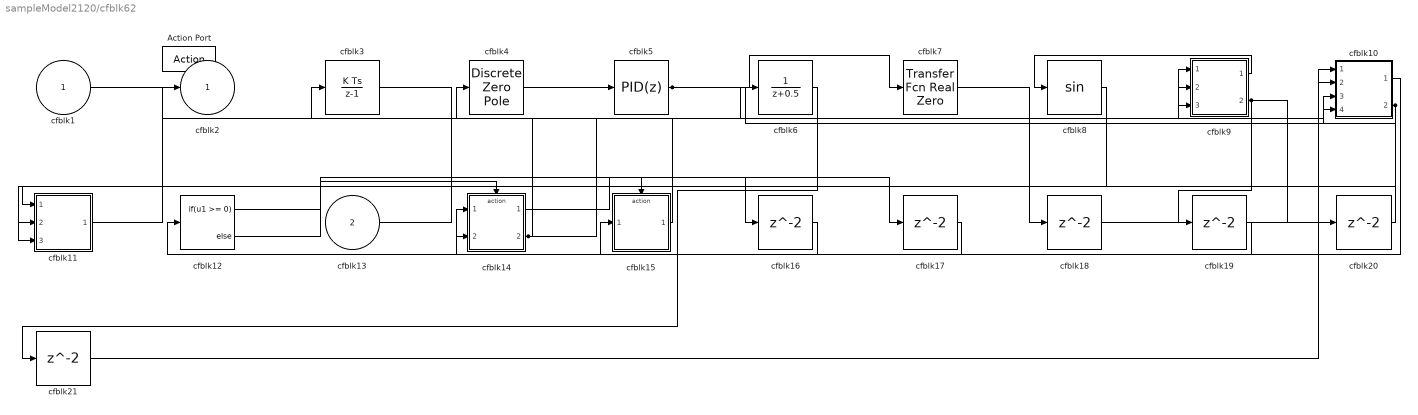
== system sampleModel2120/cfblk62 ==
  cfblk1 : Inport
  cfblk13 : Inport  Port=2
  Action Port : ActionPort  ActionPortLabel=if(u1 >= 0)
  cfblk10 : Subsystem
  cfblk11 : Subsystem
  cfblk12 : If  IfExpression=u1 >= 0  SampleTime=1
  cfblk14 : Subsystem  TreatAsAtomicUnit=on
  cfblk15 : Subsystem  TreatAsAtomicUnit=on
  cfblk{16..21} (6 alike) : Delay
  cfblk3 : DiscreteIntegrator  SampleTime=-1  ICPrevOutput=DiscIntNeverNeededParam  ICPrevScaledInput=DiscIntNeverNeededParam
  cfblk4 : DiscreteZeroPole  Poles=[0 0.5]  Gain=1  SampleTime=-1
  cfblk5 : pid_lib/PID Controller  Controller=PID  Form=Parallel  TimeDomain=Discrete-time  UseExternalTs=off  SampleTime=-1  IntegratorMethod=Forward Euler  FilterMethod=Forward Euler  ControllerParametersSource=internal  P=1  I=1  D=0  UseFilter=on  N=100  TunerSelectOption=Transfer Function Based (PID Tuner App)  InitialConditionSource=internal  InitialConditionForIntegrator=0  InitialConditionForFilter=0  DifferentiatorICPrevScaledInput=0  ExternalReset=none  TrackingMode=off  Kt=1  LimitOutput=off  SatLimitsSource=internal  UpperSaturationLimit=inf  LowerSaturationLimit=-inf  LinearizeAsGain=off  AntiWindupMode=none  Kb=1  POutMin=[]  POutMax=[]  IOutMin=[]  IOutMax=[]  DOutMin=[]  DOutMax=[]  NOutMin=[]  NOutMax=[]  SumOutMin=[]  SumOutMax=[]  SaturationOutMin=[]  SaturationOutMax=[]  PParamMin=[]  PParamMax=[]  IParamMin=[]  IParamMax=[]  DParamMin=[]  DParamMax=[]  NParamMin=[]  NParamMax=[]  KbParamMin=[]  KbParamMax=[]  KtParamMin=[]  KtParamMax=[]  KbOutMin=[]  KbOutMax=[]  KtOutMin=[]  KtOutMax=[]  IntegratorOutMin=[]  IntegratorOutMax=[]  FilterOutMin=[]  FilterOutMax=[]  SumI1OutMin=[]  SumI1OutMax=[]  SumI2OutMin=[]  SumI2OutMax=[]  SumI3OutMin=[]  SumI3OutMax=[]  SumI4OutMin=[]  SumI4OutMax=[]  SumDOutMin=[]  SumDOutMax=[]  DifferentiatorOutMin=[]  DifferentiatorOutMax=[]  FilterDiffOutCoefMin=[]  FilterDiffOutCoefMax=[]  ReciprocalOutMin=[]  ReciprocalOutMax=[]  SumDenOutMin=[]  SumDenOutMax=[]  SumNumOutMin=[]  SumNumOutMax=[]  DivideOutMin=[]  DivideOutMax=[]  UdiffTsProdOutMin=[]  UdiffTsProdOutMax=[]  NTsProdOutMin=[]  NTsProdOutMax=[]  UintegralTsProdOutMin=[]  UintegralTsProdOutMax=[]  UngainTsProdOutMin=[]  UngainTsProdOutMax=[]  IntegratorContinuousStateAttributes=''  IntegratorStateMustResolveToSignalObject=off  IntegratorRTWStateStorageClass=Auto  FilterContinuousStateAttributes=''  FilterStateMustResolveToSignalObject=off  FilterRTWStateStorageClass=Auto  ParallelPVariant=InternalParameters  IdealPVariant=Disabled  IVariant=InternalParameters  DVariant=InternalParameters  IntegratorVariant=Discrete  SatVariant=Disabled  AWVariant=Passthrough  PCopyVariant=Disabled  TRVariant=Disabled  FdbkBlocksVariant=Forward  IdealPFdbkVariant=Disabled  SatFdbkVariant=Disabled  DerivativeFilterVariant=ForwardEulerFilter  NVariant=InternalParameters  NCopyVariant=Disabled  FilterICVariant=InternalICsFilter  IntegratorICVariant=InternalICs  ExternalResetVariant=Disabled  TRSumVariant=Passthrough  SumFdbkVariant=Disabled  SumVariant=Sum_PID  TsampFilterVariant=InternalTs  TsampNgainVariant=Passthrough  TsampIntegralVariant=Passthrough  ExternalSaturationOutDataTypeStr=Inherit: Same as second input
  cfblk6 : DiscreteTransferFcn
  cfblk7 : simulink/Discrete/Transfer Fcn Real Zero  ZeroZ=0.75  ICPrevInput=0.0  DoSatur=off
      settings: SourceProductBaseCode=SL
  cfblk8 : Trigonometry
  cfblk9 : Subsystem
  cfblk2 : Outport
  wires:
  cfblk15/1(cfblk2) -> cfblk3/1
  cfblk5/1 -> cfblk7/1, cfblk9/3(cfblk11)
  cfblk10/1(cfblk2) -> cfblk14/1(cfblk1)
  cfblk14/2(cfblk8) -> cfblk4/1, cfblk9/2(cfblk10)
  cfblk8/1 -> cfblk11/1(cfblk1)
  cfblk11/1(cfblk2) -> cfblk2/1
  cfblk9/1(cfblk2) -> cfblk8/1
  cfblk9/2(cfblk12) -> cfblk11/3(cfblk8), cfblk19/1, cfblk20/1
  cfblk13/1 -> cfblk9/1(cfblk1)
  cfblk4/1 -> cfblk5/1
  cfblk1/1 -> cfblk10/3(cfblk12)
  cfblk10/2(cfblk14) -> cfblk6/1, cfblk11/2(cfblk7)
  cfblk12/1 -> cfblk14/Action
  cfblk12/2 -> cfblk15/Action
  cfblk14/1(cfblk2) -> cfblk16/1
  cfblk16/1 -> cfblk12/1
  cfblk3/1 -> cfblk17/1
  cfblk17/1 -> cfblk14/2(cfblk7)
  cfblk7/1 -> cfblk18/1
  cfblk18/1 -> cfblk10/1(cfblk1)
  cfblk19/1 -> cfblk15/1(cfblk1)
  cfblk20/1 -> cfblk10/4(cfblk13)
  cfblk6/1 -> cfblk21/1
  cfblk21/1 -> cfblk10/2(cfblk11)

== system sampleModel2120/cfblk63 ==
  cfblk1 : Inport
  Action Port : ActionPort  ActionPortLabel=else
  cfblk10 : Delay
  cfblk11 : DataTypeConversion
  cfblk12 : DataTypeConversion
  cfblk3 : DiscreteFilter
  cfblk4 : Delay  DelayLengthSource=Input port
      settings: InputPortMap=u0,p1
  cfblk5 : Sin  TimeSource=Use external signal  SampleTime=0
  cfblk6 : PermuteDimensions
  cfblk7 : Subsystem
  cfblk9 : Delay
  cfblk2 : Outport
  cfblk8 : Outport  Port=2
  wires:
  cfblk5/1 -> cfblk8/1
  cfblk1/1 -> cfblk5/1, cfblk7/3(cfblk10)
  cfblk6/1 -> cfblk4/2, cfblk9/1
  cfblk7/2(cfblk11) -> cfblk2/1
  cfblk7/3(cfblk12) -> cfblk4/1
  cfblk9/1 -> cfblk7/2(cfblk9)
  cfblk4/1 -> cfblk10/1
  cfblk10/1 -> cfblk7/1(cfblk1)
  cfblk3/1 -> cfblk11/1
  cfblk11/1 -> cfblk6/1
  cfblk7/1(cfblk2) -> cfblk12/1
  cfblk12/1 -> cfblk3/1

== system sampleModel2120/cfblk45/cfblk10 ==
  cfblk1 : Inport
  cfblk10 : Sum  Inputs=+
  cfblk11 : Bias  Bias=[143732452.396222]
  cfblk3 : DiscreteFir  SampleTime=1
  cfblk4 : simulink/Discrete/Transfer Fcn Real Zero  ZeroZ=0.75  ICPrevInput=0.0  DoSatur=off
      settings: SourceProductBaseCode=SL
  cfblk5 : simulink/Discrete/Transfer Fcn First Order  PoleZ=0.95  ICPrevOutput=0.0  DoSatur=off
  cfblk6 : Delay  DelayLengthSource=Input port  SampleTime=1
      settings: InputPortMap=u0,p1
  cfblk7 : Bias  Bias=[415695908.441253]
  cfblk8 : simulink/Math Operations/Slider Gain  gain=1  low=0  high=2
  cfblk9 : Rounding
  cfblk2 : Outport
  wires:
  cfblk9/1 -> cfblk2/1
  cfblk10/1 -> cfblk6/1
  cfblk4/1 -> cfblk5/1
  cfblk6/1 -> cfblk9/1
  cfblk7/1 -> cfblk8/1
  cfblk5/1 -> cfblk10/1
  cfblk3/1 -> cfblk4/1
  cfblk8/1 -> cfblk11/1
  cfblk1/1 -> cfblk7/1
  cfblk11/1 -> cfblk6/2, cfblk3/1

== system sampleModel2120/cfblk45/cfblk11 ==
  cfblk1 : Inport
  cfblk6 : Inport  Port=2
  cfblk7 : Inport  Port=3
  cfblk8 : Inport  Port=4
  cfblk9 : Inport  Port=5
  cfblk3 : Sum  Inputs=-+
  cfblk4 : Constant  Value=[-156405987.882864]  SampleTime=1
  cfblk5 : Constant  Value=[-751982074.552397]  SampleTime=1
  cfblk2 : Outport
  cfblk10 : Outport  Port=2
  wires:
  cfblk4/1 -> cfblk10/1
  cfblk5/1 -> cfblk2/1
  cfblk8/1 -> cfblk3/1
  cfblk7/1 -> cfblk3/2

== system sampleModel2120/cfblk45/cfblk12 ==
  cfblk1 : Inport
  cfblk11 : Inport  Port=2
  cfblk10 : Constant  Value=[257671330.793710]  SampleTime=1
  cfblk12 : Delay  SampleTime=1
  cfblk3 : simulink/Discrete/Transfer Fcn First Order  PoleZ=0.95  ICPrevOutput=0.0  DoSatur=off
  cfblk4 : Delay  ShowEnablePort=on  SampleTime=1
      settings: InputPortMap=u0,e6
  cfblk5 : DiscreteFilter  SampleTime=1
  cfblk6 : Product
  cfblk7 : Sum  Inputs=--
  cfblk8 : Sum
  cfblk9 : Constant  Value=[-533370526.019482]  SampleTime=1
  cfblk2 : Outport
  wires:
  cfblk8/1 -> cfblk4/1
  cfblk5/1 -> cfblk2/1
  cfblk1/1 -> cfblk7/1, cfblk4/2
  cfblk10/1 -> cfblk3/1
  cfblk9/1 -> cfblk5/1
  cfblk11/1 -> cfblk7/2
  cfblk7/1 -> cfblk6/1
  cfblk3/1 -> cfblk8/1
  cfblk6/1 -> cfblk8/2
  cfblk4/1 -> cfblk12/1
  cfblk12/1 -> cfblk6/2

== system sampleModel2120/cfblk45/cfblk13 ==
  cfblk1 : Inport
  cfblk11 : Inport  Port=2
  cfblk12 : Inport  Port=3
  cfblk10 : Constant  Value=[408866745.308150]  SampleTime=1
  cfblk3 : Delay  DelayLengthSource=Input port  SampleTime=1
      settings: InputPortMap=u0,p1
  cfblk4 : Sqrt  SaturateOnIntegerOverflow=on
  cfblk5 : Sqrt  Operator=rSqrt  AlgorithmType=Newton-Raphson  SaturateOnIntegerOverflow=on
  cfblk6 : PermuteDimensions
  cfblk7 : Sum  Inputs=+
  cfblk8 : Sum
  cfblk9 : Constant  Value=[-458549736.263583]  SampleTime=1
  cfblk2 : Outport
  wires:
  cfblk4/1 -> cfblk2/1
  cfblk10/1 -> cfblk8/1
  cfblk7/1 -> cfblk6/1
  cfblk11/1 -> cfblk3/1
  cfblk1/1 -> cfblk8/2
  cfblk6/1 -> cfblk4/1
  cfblk3/1 -> cfblk5/1
  cfblk12/1 -> cfblk3/2
  cfblk9/1 -> cfblk7/1

== system sampleModel2120/cfblk45/cfblk14 ==
  cfblk1 : Inport
  cfblk7 : Inport  Port=2
  cfblk8 : Inport  Port=3
  cfblk3 : Delay  SampleTime=1
  cfblk4 : Delay  SampleTime=1
  cfblk5 : ComplexToRealImag
  cfblk6 : Trigonometry
  cfblk2 : Outport
  cfblk9 : Outport  Port=2
  wires:
  cfblk3/1 -> cfblk2/1
  cfblk8/1 -> cfblk9/1
  cfblk7/1 -> cfblk6/1
  cfblk6/1 -> cfblk5/1
  cfblk5/1 -> cfblk3/1
  cfblk5/2 -> cfblk4/1

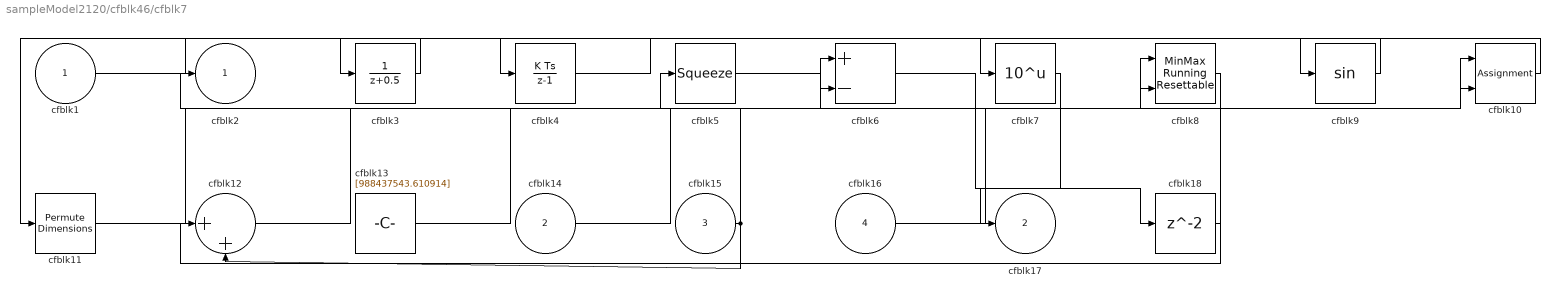
== system sampleModel2120/cfblk46/cfblk7 ==
  cfblk1 : Inport
  cfblk14 : Inport  Port=2
  cfblk15 : Inport  Port=3
  cfblk16 : Inport  Port=4
  cfblk10 : Assignment  DiagnosticForDimensions=Warning  IndexOptions=Index vector (dialog)  Indices=1  OutputSizes=1
  cfblk11 : PermuteDimensions
  cfblk12 : Sum  Inputs=|++
  cfblk13 : Constant  Value=[988437543.610914]  SampleTime=1
  cfblk18 : Delay  SampleTime=1
  cfblk3 : DiscreteTransferFcn  SampleTime=1
  cfblk4 : DiscreteIntegrator  ICPrevOutput=DiscIntNeverNeededParam  ICPrevScaledInput=DiscIntNeverNeededParam
  cfblk5 : Squeeze
  cfblk6 : Sum  Inputs=+-
  cfblk7 : Math  Operator=10^u  SaturateOnIntegerOverflow=on
  cfblk8 : simulink/Math Operations/MinMax Running Resettable  Function=min  vinit=0.0
  cfblk9 : Trigonometry
  cfblk2 : Outport
  cfblk17 : Outport  Port=2
  wires:
  cfblk10/1 -> cfblk9/1
  cfblk11/1 -> cfblk8/1
  cfblk3/1 -> cfblk11/1
  cfblk12/1 -> cfblk5/1
  cfblk1/1 -> cfblk4/1
  cfblk4/1 -> cfblk7/1
  cfblk9/1 -> cfblk3/1
  cfblk8/1 -> cfblk12/1
  cfblk13/1 -> cfblk10/1
  cfblk14/1 -> cfblk6/1
  cfblk16/1 -> cfblk10/2
  cfblk7/1 -> cfblk17/1
  cfblk15/1 -> cfblk2/1, cfblk12/2
  cfblk5/1 -> cfblk6/2
  cfblk6/1 -> cfblk18/1
  cfblk18/1 -> cfblk8/2

== system sampleModel2120/cfblk47/cfblk10 ==
  cfblk1 : Inport
  cfblk13 : Inport  Port=2
  cfblk14 : Inport  Port=3
  cfblk10 : Trigonometry
  cfblk11 : Constant  Value=[893497711.855009]  SampleTime=1
  cfblk12 : Constant  Value=[-854571024.150822]  SampleTime=1
  cfblk3 : DiscreteStateSpace
  cfblk4 : Delay  DelayLengthSource=Input port  SampleTime=1
      settings: InputPortMap=u0,p1
  cfblk5 : Rounding
  cfblk6 : Sum  Inputs=|++
  cfblk7 : DotProduct  InputSameDT=on  OutDataTypeStr=Inherit: Inherit via internal rule
  cfblk8 : Trigonometry
  cfblk9 : Product  Inputs=*
  cfblk2 : Outport
  cfblk15 : Outport  Port=2
  wires:
  cfblk12/1 -> cfblk6/1
  cfblk11/1 -> cfblk8/1
  cfblk6/1 -> cfblk9/1
  cfblk8/1 -> cfblk7/1
  cfblk4/1 -> cfblk7/2
  cfblk5/1 -> cfblk4/1
  cfblk9/1 -> cfblk2/1
  cfblk13/1 -> cfblk3/1
  cfblk10/1 -> cfblk15/1
  cfblk1/1 -> cfblk5/1
  cfblk7/1 -> cfblk10/1
  cfblk14/1 -> cfblk6/2
  cfblk3/1 -> cfblk4/2

== system sampleModel2120/cfblk47/cfblk11 ==
  cfblk1 : Inport
  cfblk11 : Delay  SampleTime=1
  cfblk12 : Delay  SampleTime=1
  cfblk3 : PermuteDimensions
  cfblk4 : Product  Inputs=*
  cfblk5 : Sin  TimeSource=Use external signal  SampleTime=0
  cfblk6 : Rounding
  cfblk7 : Sum  Inputs=+
  cfblk8 : DotProduct  InputSameDT=on  OutDataTypeStr=Inherit: Inherit via internal rule
  cfblk9 : Product
  cfblk2 : Outport
  cfblk10 : Outport  Port=2
  wires:
  cfblk5/1 -> cfblk7/1, cfblk8/1
  cfblk9/1 -> cfblk6/1
  cfblk4/1 -> cfblk10/1
  cfblk7/1 -> cfblk3/1, cfblk12/1
  cfblk8/1 -> cfblk2/1
  cfblk1/1 -> cfblk9/1
  cfblk6/1 -> cfblk8/2, cfblk11/1
  cfblk3/1 -> cfblk4/1
  cfblk11/1 -> cfblk9/2
  cfblk12/1 -> cfblk5/1

== system sampleModel2120/cfblk47/cfblk12 ==
  cfblk1 : Inport
  cfblk11 : Inport  Port=2
  cfblk12 : Inport  Port=3
  cfblk13 : Inport  Port=4
  cfblk14 : Inport  Port=5
  cfblk15 : Inport  Port=6
  cfblk10 : Rounding
  cfblk16 : Delay  SampleTime=1
  cfblk3 : DiscreteFir  SampleTime=1
  cfblk4 : DiscreteFilter  SampleTime=1
  cfblk5 : simulink/Discrete/Transfer Fcn Lead or Lag  PoleZ=0.95  ZeroZ=0.75  ICPrevOutput=0.0  ICPrevInput=0.0  DoSatur=off
      settings: SourceProductBaseCode=SL
  cfblk6 : DotProduct  InputSameDT=on  OutDataTypeStr=Inherit: Inherit via internal rule
  cfblk7 : Sqrt  SaturateOnIntegerOverflow=on
  cfblk8 : DotProduct  InputSameDT=on  OutDataTypeStr=Inherit: Inherit via internal rule
  cfblk9 : DotProduct  InputSameDT=on  OutDataTypeStr=Inherit: Inherit via internal rule
  cfblk2 : Outport
  wires:
  cfblk3/1 -> cfblk7/1
  cfblk15/1 -> cfblk2/1
  cfblk11/1 -> cfblk5/1
  cfblk7/1 -> cfblk6/1
  cfblk14/1 -> cfblk4/1
  cfblk4/1 -> cfblk8/1
  cfblk12/1 -> cfblk6/2
  cfblk6/1 -> cfblk9/1
  cfblk13/1 -> cfblk8/2
  cfblk8/1 -> cfblk9/2
  cfblk9/1 -> cfblk10/1
  cfblk10/1 -> cfblk16/1
  cfblk16/1 -> cfblk3/1

== system sampleModel2120/cfblk47/cfblk9 ==
  cfblk1 : Inport
  cfblk12 : Inport  Port=2
  cfblk13 : Inport  Port=3
  cfblk10 : DotProduct  InputSameDT=on  OutDataTypeStr=Inherit: Inherit via internal rule
  cfblk11 : Sum  Inputs=+-
  cfblk3 : pid_lib/PID Controller  Controller=PID  Form=Parallel  TimeDomain=Discrete-time  UseExternalTs=off  SampleTime=1  IntegratorMethod=Forward Euler  FilterMethod=Forward Euler  ControllerParametersSource=internal  P=1  I=1  D=0  UseFilter=on  N=100  TunerSelectOption=Transfer Function Based (PID Tuner App)  InitialConditionSource=internal  InitialConditionForIntegrator=0  InitialConditionForFilter=0  DifferentiatorICPrevScaledInput=0  ExternalReset=none  TrackingMode=off  Kt=1  LimitOutput=off  SatLimitsSource=internal  UpperSaturationLimit=inf  LowerSaturationLimit=-inf  LinearizeAsGain=off  AntiWindupMode=none  Kb=1  POutMin=[]  POutMax=[]  IOutMin=[]  IOutMax=[]  DOutMin=[]  DOutMax=[]  NOutMin=[]  NOutMax=[]  SumOutMin=[]  SumOutMax=[]  SaturationOutMin=[]  SaturationOutMax=[]  PParamMin=[]  PParamMax=[]  IParamMin=[]  IParamMax=[]  DParamMin=[]  DParamMax=[]  NParamMin=[]  NParamMax=[]  KbParamMin=[]  KbParamMax=[]  KtParamMin=[]  KtParamMax=[]  KbOutMin=[]  KbOutMax=[]  KtOutMin=[]  KtOutMax=[]  IntegratorOutMin=[]  IntegratorOutMax=[]  FilterOutMin=[]  FilterOutMax=[]  SumI1OutMin=[]  SumI1OutMax=[]  SumI2OutMin=[]  SumI2OutMax=[]  SumI3OutMin=[]  SumI3OutMax=[]  SumI4OutMin=[]  SumI4OutMax=[]  SumDOutMin=[]  SumDOutMax=[]  DifferentiatorOutMin=[]  DifferentiatorOutMax=[]  FilterDiffOutCoefMin=[]  FilterDiffOutCoefMax=[]  ReciprocalOutMin=[]  ReciprocalOutMax=[]  SumDenOutMin=[]  SumDenOutMax=[]  SumNumOutMin=[]  SumNumOutMax=[]  DivideOutMin=[]  DivideOutMax=[]  UdiffTsProdOutMin=[]  UdiffTsProdOutMax=[]  NTsProdOutMin=[]  NTsProdOutMax=[]  UintegralTsProdOutMin=[]  UintegralTsProdOutMax=[]  UngainTsProdOutMin=[]  UngainTsProdOutMax=[]  IntegratorContinuousStateAttributes=''  IntegratorStateMustResolveToSignalObject=off  IntegratorRTWStateStorageClass=Auto  FilterContinuousStateAttributes=''  FilterStateMustResolveToSignalObject=off  FilterRTWStateStorageClass=Auto  ParallelPVariant=InternalParameters  IdealPVariant=Disabled  IVariant=InternalParameters  DVariant=InternalParameters  IntegratorVariant=Discrete  SatVariant=Disabled  AWVariant=Passthrough  PCopyVariant=Disabled  TRVariant=Disabled  FdbkBlocksVariant=Forward  IdealPFdbkVariant=Disabled  SatFdbkVariant=Disabled  DerivativeFilterVariant=ForwardEulerFilter  NVariant=InternalParameters  NCopyVariant=Disabled  FilterICVariant=InternalICsFilter  IntegratorICVariant=InternalICs  ExternalResetVariant=Disabled  TRSumVariant=Passthrough  SumFdbkVariant=Disabled  SumVariant=Sum_PID  TsampFilterVariant=InternalTs  TsampNgainVariant=Passthrough  TsampIntegralVariant=Passthrough  ExternalSaturationOutDataTypeStr=Inherit: Same as second input
  cfblk4 : simulink/Discrete/Transfer Fcn Real Zero  ZeroZ=0.75  ICPrevInput=0.0  DoSatur=off
      settings: SourceProductBaseCode=SL
  cfblk5 : simulink/Discrete/Transfer Fcn Lead or Lag  PoleZ=0.95  ZeroZ=0.75  ICPrevOutput=0.0  ICPrevInput=0.0  DoSatur=off
      settings: SourceProductBaseCode=SL
  cfblk6 : simulink/Discrete/Transfer Fcn First Order  PoleZ=0.95  ICPrevOutput=0.0  DoSatur=off
  cfblk7 : ComplexToMagnitudeAngle
  cfblk8 : Rounding
  cfblk9 : Bias  Bias=[-695140496.108146]
  cfblk2 : Outport
  cfblk14 : Outport  Port=2
  wires:
  cfblk8/1 -> cfblk2/1
  cfblk7/1 -> cfblk11/1
  cfblk12/1 -> cfblk7/1
  cfblk6/1 -> cfblk9/1
  cfblk13/1 -> cfblk3/1
  cfblk5/1 -> cfblk10/1
  cfblk3/1 -> cfblk6/1
  cfblk1/1 -> cfblk10/2
  cfblk9/1 -> cfblk8/1
  cfblk10/1 -> cfblk14/1
  cfblk4/1 -> cfblk11/2
  cfblk11/1 -> cfblk5/1
  cfblk7/2 -> cfblk4/1

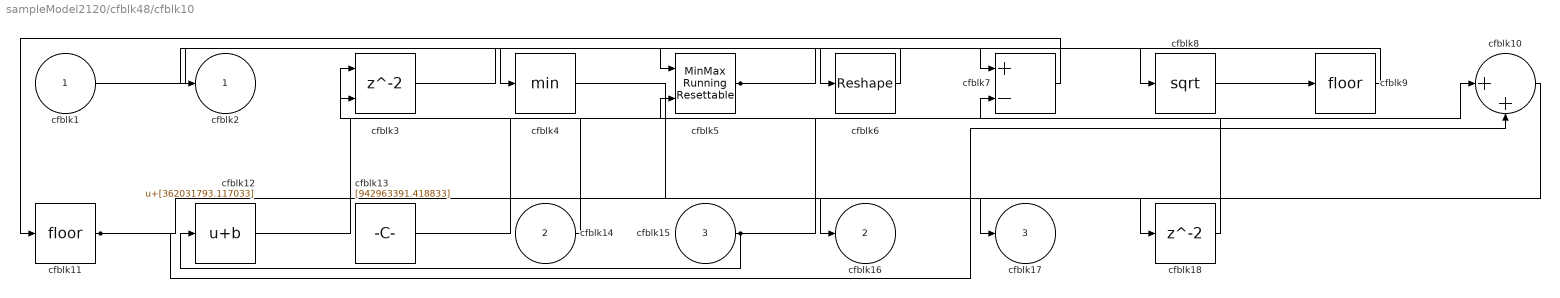
== system sampleModel2120/cfblk48/cfblk10 ==
  cfblk1 : Inport
  cfblk14 : Inport  Port=2
  cfblk15 : Inport  Port=3
  cfblk10 : Sum  Inputs=|++
  cfblk11 : Rounding
  cfblk12 : Bias  Bias=[362031793.117033]
  cfblk13 : Constant  Value=[942963391.418833]  SampleTime=1
  cfblk18 : Delay  SampleTime=1
  cfblk3 : Delay  ShowEnablePort=on  SampleTime=1
      settings: InputPortMap=u0,e6
  cfblk4 : MinMax
  cfblk5 : simulink/Math Operations/MinMax Running Resettable  Function=min  vinit=0.0
  cfblk6 : Reshape
  cfblk7 : Sum  Inputs=+-
  cfblk8 : Sqrt  SaturateOnIntegerOverflow=on
  cfblk9 : Rounding
  cfblk2 : Outport
  cfblk16 : Outport  Port=2
  cfblk17 : Outport  Port=3
  wires:
  cfblk1/1 -> cfblk4/1
  cfblk8/1 -> cfblk9/1
  cfblk10/1 -> cfblk17/1
  cfblk13/1 -> cfblk10/1
  cfblk6/1 -> cfblk5/1
  cfblk15/1 -> cfblk12/1, cfblk7/2
  cfblk7/1 -> cfblk11/1
  cfblk3/1 -> cfblk6/1
  cfblk11/1 -> cfblk10/2, cfblk18/1
  cfblk14/1 -> cfblk3/1
  cfblk4/1 -> cfblk16/1
  cfblk5/1 -> cfblk7/1, cfblk8/1
  cfblk9/1 -> cfblk2/1
  cfblk12/1 -> cfblk5/2
  cfblk18/1 -> cfblk3/2

== system sampleModel2120/cfblk48/cfblk11 ==
  cfblk1 : Inport
  cfblk7 : Inport  Port=2
  cfblk8 : Inport  Port=3
  cfblk9 : Inport  Port=4
  cfblk10 : Inport  Port=5
  cfblk3 : pid_lib/PID Controller  Controller=PID  Form=Parallel  TimeDomain=Discrete-time  UseExternalTs=off  SampleTime=1  IntegratorMethod=Forward Euler  FilterMethod=Forward Euler  ControllerParametersSource=internal  P=1  I=1  D=0  UseFilter=on  N=100  TunerSelectOption=Transfer Function Based (PID Tuner App)  InitialConditionSource=internal  InitialConditionForIntegrator=0  InitialConditionForFilter=0  DifferentiatorICPrevScaledInput=0  ExternalReset=none  TrackingMode=off  Kt=1  LimitOutput=off  SatLimitsSource=internal  UpperSaturationLimit=inf  LowerSaturationLimit=-inf  LinearizeAsGain=off  AntiWindupMode=none  Kb=1  POutMin=[]  POutMax=[]  IOutMin=[]  IOutMax=[]  DOutMin=[]  DOutMax=[]  NOutMin=[]  NOutMax=[]  SumOutMin=[]  SumOutMax=[]  SaturationOutMin=[]  SaturationOutMax=[]  PParamMin=[]  PParamMax=[]  IParamMin=[]  IParamMax=[]  DParamMin=[]  DParamMax=[]  NParamMin=[]  NParamMax=[]  KbParamMin=[]  KbParamMax=[]  KtParamMin=[]  KtParamMax=[]  KbOutMin=[]  KbOutMax=[]  KtOutMin=[]  KtOutMax=[]  IntegratorOutMin=[]  IntegratorOutMax=[]  FilterOutMin=[]  FilterOutMax=[]  SumI1OutMin=[]  SumI1OutMax=[]  SumI2OutMin=[]  SumI2OutMax=[]  SumI3OutMin=[]  SumI3OutMax=[]  SumI4OutMin=[]  SumI4OutMax=[]  SumDOutMin=[]  SumDOutMax=[]  DifferentiatorOutMin=[]  DifferentiatorOutMax=[]  FilterDiffOutCoefMin=[]  FilterDiffOutCoefMax=[]  ReciprocalOutMin=[]  ReciprocalOutMax=[]  SumDenOutMin=[]  SumDenOutMax=[]  SumNumOutMin=[]  SumNumOutMax=[]  DivideOutMin=[]  DivideOutMax=[]  UdiffTsProdOutMin=[]  UdiffTsProdOutMax=[]  NTsProdOutMin=[]  NTsProdOutMax=[]  UintegralTsProdOutMin=[]  UintegralTsProdOutMax=[]  UngainTsProdOutMin=[]  UngainTsProdOutMax=[]  IntegratorContinuousStateAttributes=''  IntegratorStateMustResolveToSignalObject=off  IntegratorRTWStateStorageClass=Auto  FilterContinuousStateAttributes=''  FilterStateMustResolveToSignalObject=off  FilterRTWStateStorageClass=Auto  ParallelPVariant=InternalParameters  IdealPVariant=Disabled  IVariant=InternalParameters  DVariant=InternalParameters  IntegratorVariant=Discrete  SatVariant=Disabled  AWVariant=Passthrough  PCopyVariant=Disabled  TRVariant=Disabled  FdbkBlocksVariant=Forward  IdealPFdbkVariant=Disabled  SatFdbkVariant=Disabled  DerivativeFilterVariant=ForwardEulerFilter  NVariant=InternalParameters  NCopyVariant=Disabled  FilterICVariant=InternalICsFilter  IntegratorICVariant=InternalICs  ExternalResetVariant=Disabled  TRSumVariant=Passthrough  SumFdbkVariant=Disabled  SumVariant=Sum_PID  TsampFilterVariant=InternalTs  TsampNgainVariant=Passthrough  TsampIntegralVariant=Passthrough  ExternalSaturationOutDataTypeStr=Inherit: Same as second input
  cfblk4 : simulink/Discrete/Transfer Fcn Real Zero  ZeroZ=0.75  ICPrevInput=0.0  DoSatur=off
      settings: SourceProductBaseCode=SL
  cfblk5 : simulink/Discrete/Transfer Fcn First Order  PoleZ=0.95  ICPrevOutput=0.0  DoSatur=off
  cfblk6 : simulink/Discrete/Transfer Fcn Lead or Lag  PoleZ=0.95  ZeroZ=0.75  ICPrevOutput=0.0  ICPrevInput=0.0  DoSatur=off
      settings: SourceProductBaseCode=SL
  cfblk2 : Outport
  cfblk11 : Outport  Port=2
  wires:
  cfblk9/1 -> cfblk5/1
  cfblk1/1 -> cfblk11/1
  cfblk10/1 -> cfblk3/1
  cfblk6/1 -> cfblk2/1
  cfblk5/1 -> cfblk6/1
  cfblk7/1 -> cfblk4/1

== system sampleModel2120/cfblk48/cfblk12 ==
  cfblk1 : Inport
  cfblk8 : Inport  Port=2
  cfblk9 : Inport  Port=3
  cfblk3 : Sin  TimeSource=Use external signal  SampleTime=0
  cfblk4 : Trigonometry
  cfblk5 : Abs
  cfblk6 : Constant  Value=[518719100.670352]  SampleTime=1
  cfblk7 : Constant  Value=[188716034.408801]  SampleTime=1
  cfblk2 : Outport
  cfblk10 : Outport  Port=2
  wires:
  cfblk8/1 -> cfblk10/1
  cfblk6/1 -> cfblk4/1
  cfblk9/1 -> cfblk2/1
  cfblk4/1 -> cfblk5/1
  cfblk5/1 -> cfblk3/1

== system sampleModel2120/cfblk49/cfblk5 ==
  cfblk1 : Inport
  cfblk7 : Inport  Port=2
  cfblk3 : ComplexToRealImag
  cfblk4 : Sqrt  Operator=rSqrt  AlgorithmType=Newton-Raphson  SaturateOnIntegerOverflow=on
  cfblk5 : Rounding
  cfblk6 : Reshape
  cfblk8 : Delay  SampleTime=1
  cfblk2 : Outport
  wires:
  cfblk3/1 -> cfblk4/1
  cfblk6/1 -> cfblk5/1
  cfblk1/1 -> cfblk6/1
  cfblk3/2 -> cfblk2/1
  cfblk4/1 -> cfblk8/1
  cfblk8/1 -> cfblk3/1
